simulink model "EPD629_WilliamsJ_Project_"  (R2021b)
settings: Solver=VariableStepAuto  StartTime=0.0  StopTime=StopTime  MaxStep=0.005  RelTol=1e-4
values from neighbouring files (symbols this model uses):
  AxleRatio = 11.47    [ProjectScript.m]
  BrakeDrag_N = 2.5    [ProjectScript.m]
  CableStrokeVsPedalPos_mmpdeg = 0.995519    [ProjectScript.m]
  Cd = 0.7691142    [ProjectScript.m]
  Crr = 0.0138796    [ProjectScript.m]
  CTireRollRadius = 0.944    [ProjectScript.m]
  CVTEngagementSpd_rpm = 1400    [ProjectScript.m]
  CVTRatioCoeffVsMphA = 0.000494471902965804    (= 0.000494471902966)    [ProjectScript.m]
  CVTRatioCoeffVsMphB = -0.0203171948865201    (= -0.0203171948865)    [ProjectScript.m]
  CVTRatioCoeffVsMphC = 0.301637634575451    (= 0.301637634575)    [ProjectScript.m]
  CVTRatioCoeffVsMphD = -2.09463337350964    (= -2.09463337351)    [ProjectScript.m]
  CVTRatioCoeffVsMphE = 7.47628950179633    (= 7.4762895018)    [ProjectScript.m]
  DistCableSinkThrottle_mm = 0.25    [ProjectScript.m]
  EngPowerTableData_hp = [0, 0, 0, 0, 0 ... (first row only)    [ProjectScript.m]
  EngPowerTableSpdBreakpoints_rpm = (0:500:7500)    [ProjectScript.m]
  EngPowerTableThrottleBreakpoints_prcnt = [0:.25:1]    [ProjectScript.m]
  FlyCoeffAClosed = 5.31512605042017e-8    (= 5.31512605042e-08)    [ProjectScript.m]
  FlyCoeffAOpen = 2.27450980392157e-7    (= 2.27450980392e-07)    [ProjectScript.m]
  FlyCoeffBClosed = 0.0000162815126050419    (= 1.6281512605e-05)    [ProjectScript.m]
  FlyCoeffBOpen = -0.000070868347338936    (= -7.08683473389e-05)    [ProjectScript.m]
  FlyCoeffCClosed = -0.0102941176470588    (= -0.0102941176471)    [ProjectScript.m]
  FlyCoeffCOpen = 0.00588235294117689    (= 0.00588235294118)    [ProjectScript.m]
  g = 9.80665    [ProjectScript.m]
  GearboxRatio = 1.95    [ProjectScript.m]
  GovArmRange_deg = 14.7    [ProjectScript.m]
  GradeIncline_pcnt = 0    [ProjectScript.m]
  LengthGovArmLower_mm = 90.4    [ProjectScript.m]
  LengthGovArmUpper_mm = 67.5    [ProjectScript.m]
  MassVehicle_kg = (CurbWeight_lbm + VehiclePayload_lbm)*0.4535924    (= 589.67012)    [ProjectScript.m]
  PedalPosMax_deg = 30    [ProjectScript.m]
  PedalTravelIntTension_deg = 10    [ProjectScript.m]
  rho_air = 1.224991    [ProjectScript.m]
  SpringRate_lbfpin = 12.6    [ProjectScript.m]
  ThrottleCableDia_mm = 1.190625    [ProjectScript.m]
  ThrottleLeverArmRadius_mm = 14.25    [ProjectScript.m]
  ThrottlePosMax_deg = 82    [ProjectScript.m]
  ThrottleReturnSpringPreload_Nmm = 163.7711    [ProjectScript.m]
  ThrottleReturnSpringRate_Nmmpdeg = 0.786881    [ProjectScript.m]
  TireDia_in = 18    [ProjectScript.m]
  VehicleFrontalArea_m2 = 1.8    [ProjectScript.m]
undefined symbols (not defined in the file or in its folder): CaptureTime, DesCruisingSpeed_mph, GovernorSet, Pedal_Change_After_Dyno
libraries: simulink x7, simulink_extras x2
settings Model: Creator=jwilli42  LastModifiedBy=jwilli42
settings OptimizationCC: BlockReduction=off  DefaultParameterBehavior=Inlined  BufferReuse=off
settings DebuggingCC: AlgebraicLoopMsg=none

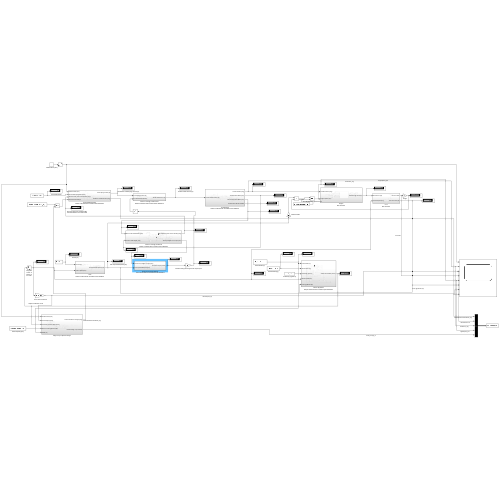
[thumbnail: Simulink's stored preview of the top-level diagram]
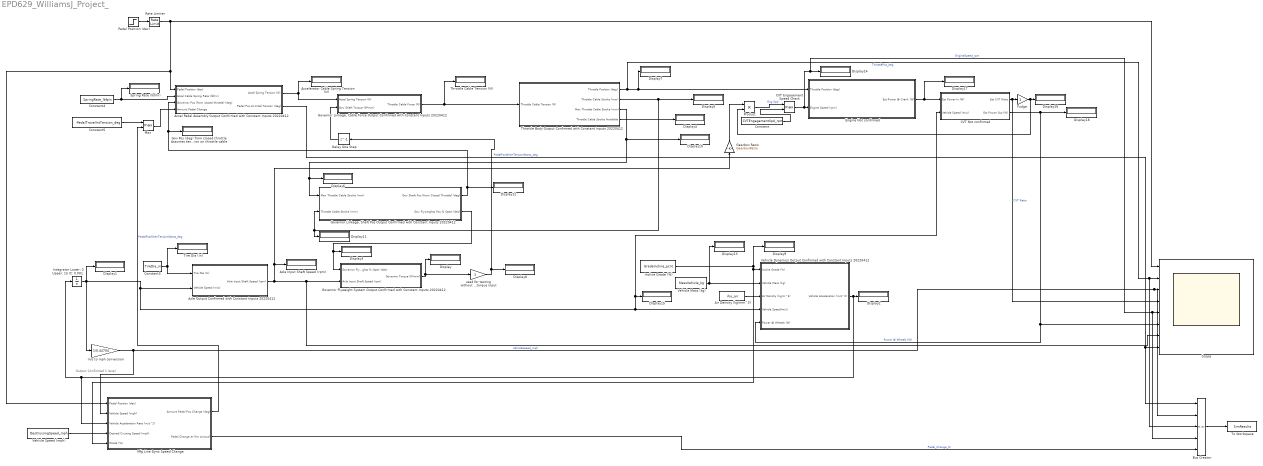
== system EPD629_WilliamsJ_Project_ ==
  note: Output Confirmed 1 level
  Accel Pedal Assembly Output Confirmed with Constant Inputs 20220412 : Subsystem
  Accelerator Cable Spring Tension (N) : Display
  Air Density (kg/mm^3) : Constant  Value=rho_air
  Axle Output Confirmed with Constant Inputs 20220412 : Subsystem
  Axle Input Shaft Speed (rpm) : Display
  Bus Creator : BusCreator  Inputs=5
  CVT Not confirmed : Subsystem
  CVT Engagement Speed Check : MinMax  Function=max  Inputs=2
  Constant : Constant  Value=CVTEngagementSpd_rpm
  Constant3 : Constant  Value=TireDia_in
  Constant4 : Constant  Value=SpringRate_lbfpin
  Constant5 : Constant  Value=-PedalTravelIntTension_deg
  Delay One Step : Delay  DelayLength=1
  Display{,1..18} (19 alike) : Display
  Engine Not confirmed : Subsystem
  Fudge : Gain
  Gearbox Ratio : Gain  Gain=GearboxRatio
  Gov Pos (deg) from closed throttle Assumes tension on throttle cable : Display
  Governor Flyweight System Output Confirmed with Constant Inputs 20220412 : Subsystem
  "Governor Linkage, Cable Force Output Confirmed with Constant Inputs 20220412" : Subsystem
  "Governor Linkage, Shaft Pos Output Confirmed with Constant Inputs 20220412" : Subsystem
  Incline Grade (%) : Constant  Value=GradeIncline_pcnt
  "Integrator Lower: 0 Upper: 15 IC: 0.001 " : Integrator  InitialCondition=.1  LimitOutput=on  UpperSaturationLimit=15  LowerSaturationLimit=0
  Max : MinMax  Function=max  Inputs=2
  Mfg Line Dyno Speed Change : Subsystem
  Pedal Position (dec) : Step  Time=0.5  SampleTime=0
  Product : Product
  Rate Limiter : RateLimiter  RisingSlewLimit=20  FallingSlewLimit=-30  SampleTimeMode=inherited
  Scope : Scope  NumInputPorts=8
  Spring Rate (lbf/in) : Display
  Throttle Body Output Confirmed with Constant Inputs 20220412 : Subsystem
  "Throttle Cable Tension (N) " : Display
  Tire Dia (in) : Display
  To Workspace : ToWorkspace  VariableName=SimResults  SaveFormat=Timeseries  SampleTime=-1
      settings: MaxDataPoints=1
  "Vehicle Dynamics Output Confirmed with Constant Inputs 20220412 " : Subsystem
  Vehicle Mass (kg) : Constant  Value=MassVehicle_kg
  Vehicle Speed (mph) : Constant  Value=DesCruisingSpeed_mph
  m/s to mph conversion : Gain  Gain=1/0.44704
  used for testing without governor torque input : Gain
  wires:
  Vehicle Mass (kg)/1 -> "Vehicle Dynamics Output Confirmed with Constant Inputs 20220412 "/2(Vehicle Mass (kg)), Display13/1
  Air Density (kg/mm^3)/1 -> "Vehicle Dynamics Output Confirmed with Constant Inputs 20220412 "/3(Air Density (kg/m^3))
  Vehicle Speed (mph)/1 -> Mfg Line Dyno Speed Change/4(Desired Cruising Speed (mph))
  Constant3/1 -> Tire Dia (in)/1, Axle Output Confirmed with Constant Inputs 20220412/1(Tire Dia (In))
  Throttle Body Output Confirmed with Constant Inputs 20220412/3(Max Throttle Cable Stroke (mm)) -> Display10/1, "Governor Linkage, Shaft Pos Output Confirmed with Constant Inputs 20220412"/1(Max Throttle Cable Stroke (mm)), Display6/1
  Axle Output Confirmed with Constant Inputs 20220412/1(Axle Input Shaft Speed (rpm)) -> Axle Input Shaft Speed (rpm)/1, Gearbox Ratio/1, Scope/7, Governor Flyweight System Output Confirmed with Constant Inputs 20220412/2(Axle Input Shaft Speed (rpm))
  Constant4/1 -> Accel Pedal Assembly Output Confirmed with Constant Inputs 20220412/2(Accel Cable Spring Rate (lbf/in)), Spring Rate (lbf/in)/1
  Pedal Position (dec)/1 -> Rate Limiter/1
  Throttle Body Output Confirmed with Constant Inputs 20220412/1(Throttle Position (deg)) -> Scope/2, Bus Creator/3, Engine Not confirmed/1(Throttle Position (deg)), Display7/1  "ThrottlePos_deg"
  Throttle Body Output Confirmed with Constant Inputs 20220412/4(Throttle Cable Stroke Available) -> Display4/1
  Engine Not confirmed/1(Est Power @ Crank (W)) -> Display17/1, CVT Not confirmed/1(Est Power In (W))
  Gearbox Ratio/1 -> Product/1
  CVT Not confirmed/1(Est CVT Ratio) -> Scope/4, Fudge/1  "CVT Ratio"
  Fudge/1 -> Display16/1, Product/2
  CVT Not confirmed/2(Est Power Out (W)) -> "Vehicle Dynamics Output Confirmed with Constant Inputs 20220412 "/5(Power @ Wheels (W)), Scope/6, Display18/1  "Power @ Wheels (W)"
  m/s to mph conversion/1 -> Bus Creator/2, Scope/3, Mfg Line Dyno Speed Change/2(Vehicle Speed (mph))  "VehicleSpeed_mph"
  Product/1 -> CVT Engagement Speed Check/1  "Eng Spd"
  Constant/1 -> CVT Engagement Speed Check/2
  Governor Flyweight System Output Confirmed with Constant Inputs 20220412/1(Governor Torque (N*mm)) -> Display/1, used for testing without governor torque input/1
  CVT Engagement Speed Check/1 -> Scope/5, Bus Creator/4, Display14/1, Engine Not confirmed/2(Engine Speed (rpm))  "EngineSpeed_rpm"
  Rate Limiter/1 -> Mfg Line Dyno Speed Change/1(Pedal Position (dec)), Accel Pedal Assembly Output Confirmed with Constant Inputs 20220412/1(Pedal Position (dec)), Scope/1
  Mfg Line Dyno Speed Change/1(Amount Pedal Pos Change (deg)) -> Max/2  "PedalPosWhenTensionStarts_deg"
  Incline Grade (%)/1 -> Mfg Line Dyno Speed Change/5(Grade (%)), "Vehicle Dynamics Output Confirmed with Constant Inputs 20220412 "/1(Incline Grade (%)), Display9/1
  Constant5/1 -> Max/1
  Max/1 -> Accel Pedal Assembly Output Confirmed with Constant Inputs 20220412/4(Amount Pedal Change)
  Accel Pedal Assembly Output Confirmed with Constant Inputs 20220412/2(Pedal Pos at Initial Tension (deg)) -> Scope/8, Bus Creator/1  "PedalPosWhenTensionStarts_deg"
  Mfg Line Dyno Speed Change/2(Pedal Change Itr (for simout)) -> Bus Creator/5  "Pedal_Change_Itr"
  Bus Creator/1 -> To Workspace/1
  used for testing without governor torque input/1 -> Delay One Step/1, Display8/1
  "Vehicle Dynamics Output Confirmed with Constant Inputs 20220412 "/1(Vehicle Acceleration (m/s^2)) -> Mfg Line Dyno Speed Change/3(Vehicle Acceleration Rate (m/s^2)), "Integrator Lower: 0 Upper: 15 IC: 0.001 "/1, Display2/1
  Delay One Step/1 -> "Governor Linkage, Cable Force Output Confirmed with Constant Inputs 20220412"/2(Gov Shaft Torque (N*mm))
  Accel Pedal Assembly Output Confirmed with Constant Inputs 20220412/1(Accel Spring Tension (N)) -> "Governor Linkage, Cable Force Output Confirmed with Constant Inputs 20220412"/1(Accel Spring Tension (N)), Accelerator Cable Spring Tension (N)/1
  "Integrator Lower: 0 Upper: 15 IC: 0.001 "/1 -> m/s to mph conversion/1, CVT Not confirmed/2(Vehicle Speed (m/s)), Display15/1, "Vehicle Dynamics Output Confirmed with Constant Inputs 20220412 "/4(Vehicle Speed(m/s)), Axle Output Confirmed with Constant Inputs 20220412/2(Vehicle Speed (m/s)), Display1/1
  "Governor Linkage, Shaft Pos Output Confirmed with Constant Inputs 20220412"/2(Gov Flyweights Pos % Open (dec)) -> Governor Flyweight System Output Confirmed with Constant Inputs 20220412/1(Governor Flyweights % Open (dec)), Display3/1
  "Governor Linkage, Cable Force Output Confirmed with Constant Inputs 20220412"/1(Throttle Cable Force (N)) -> Throttle Body Output Confirmed with Constant Inputs 20220412/1(Throttle Cable Tension (N)), "Throttle Cable Tension (N) "/1
  "Governor Linkage, Shaft Pos Output Confirmed with Constant Inputs 20220412"/1(Gov Shaft Pos (from Closed Throttle) (deg)) -> Accel Pedal Assembly Output Confirmed with Constant Inputs 20220412/3(Governor Pos (from closed throttle) (deg)), Gov Pos (deg) from closed throttle Assumes tension on throttle cable/1, Display12/1
  Throttle Body Output Confirmed with Constant Inputs 20220412/2(Throttle Cable Stroke (mm)) -> "Governor Linkage, Shaft Pos Output Confirmed with Constant Inputs 20220412"/2(Throttle Cable Stroke (mm)), Display11/1, Display5/1

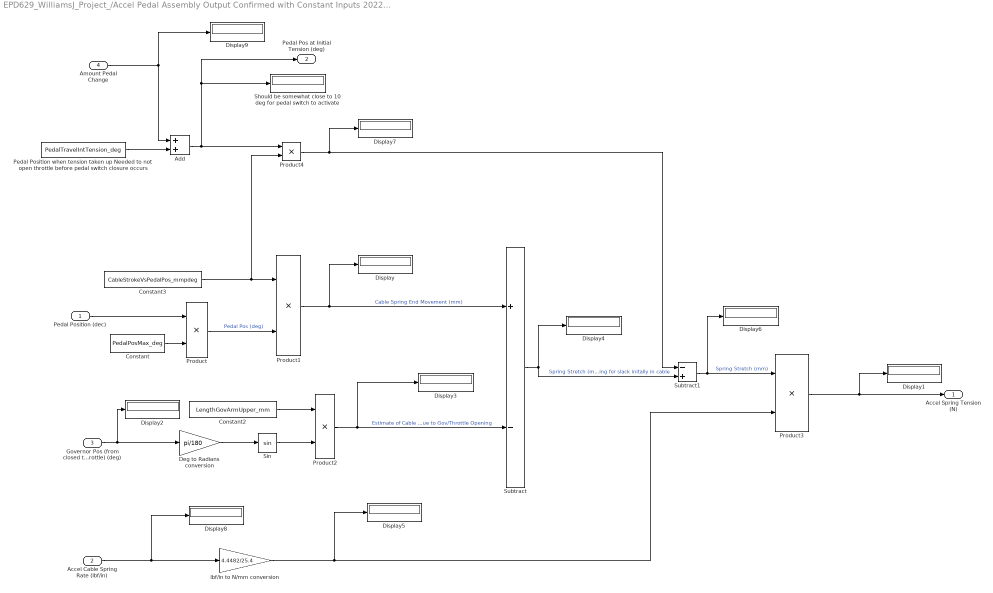
== system EPD629_WilliamsJ_Project_/Accel Pedal Assembly Output Confirmed with Constant Inputs 20220412 ==
  Pedal Position (dec) : Inport
  Accel Cable Spring Rate (lbf/in) : Inport  Port=2
  Governor Pos (from closed throttle) (deg) : Inport  Port=3
  Amount Pedal Change : Inport  Port=4
  Add : Sum
  Constant : Constant  Value=PedalPosMax_deg
  Constant2 : Constant  Value=LengthGovArmUpper_mm
  Constant3 : Constant  Value=CableStrokeVsPedalPos_mmpdeg
  Deg to Radians conversion : Gain  Gain=pi/180
  Display{,1..9} (10 alike) : Display
  Pedal Position when tension taken up Needed to not open throttle before pedal switch closure occurs : Constant  Value=PedalTravelIntTension_deg
  Product{,1..4} (5 alike) : Product
  Should be somewhat close to 10 deg for pedal switch to activate : Display
  Sin : Trigonometry
  Subtract : Sum  Inputs=+-
  Subtract1 : Sum  Inputs=-+
  lbf/in to N/mm conversion : Gain  Gain=4.4482/25.4
  Accel Spring Tension (N) : Outport
  Pedal Pos at Initial Tension (deg) : Outport  Port=2
  wires:
  Constant/1 -> Product/2
  Product/1 -> Product1/2  "Pedal Pos (deg)"
  Governor Pos (from closed throttle) (deg)/1 -> Display2/1, Deg to Radians conversion/1
  Deg to Radians conversion/1 -> Sin/1
  Sin/1 -> Product2/2
  Constant2/1 -> Product2/1
  Product1/1 -> Display/1, Subtract/1  "Cable Spring End Movement (mm)"
  Product2/1 -> Display3/1, Subtract/2  "Estimate of Cable Travel Due to Gov/Throttle Opening"
  lbf/in to N/mm conversion/1 -> Display5/1, Product3/2
  Subtract/1 -> Subtract1/2, Display4/1  "Spring Stretch (mm) w/out accounting for slack initally in cable"
  Product3/1 -> Display1/1, Accel Spring Tension (N)/1
  Accel Cable Spring Rate (lbf/in)/1 -> Display8/1, lbf/in to N/mm conversion/1
  Product4/1 -> Subtract1/1, Display7/1
  Subtract1/1 -> Product3/1, Display6/1  "Spring Stretch (mm)"
  Pedal Position (dec)/1 -> Product/1
  Pedal Position when tension taken up Needed to not open throttle before pedal switch closure occurs/1 -> Add/2
  Constant3/1 -> Product1/1, Product4/2
  Add/1 -> Pedal Pos at Initial Tension (deg)/1, Should be somewhat close to 10 deg for pedal switch to activate/1, Product4/1
  Amount Pedal Change/1 -> Add/1, Display9/1

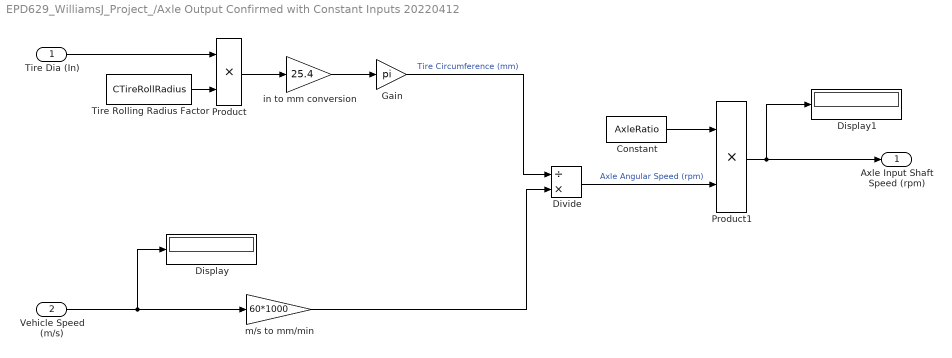
== system EPD629_WilliamsJ_Project_/Axle Output Confirmed with Constant Inputs 20220412 ==
  Tire Dia (In) : Inport
  Vehicle Speed (m/s) : Inport  Port=2
  Constant : Constant  Value=AxleRatio
  Display : Display
  Display1 : Display
  Divide : Product  Inputs=/*
  Gain : Gain  Gain=pi
  Product : Product
  Product1 : Product
  Tire Rolling Radius Factor : Constant  Value=CTireRollRadius
  in to mm conversion : Gain  Gain=25.4
  m/s to mm/min : Gain  Gain=60*1000
  Axle Input Shaft Speed (rpm) : Outport
  wires:
  Tire Rolling Radius Factor/1 -> Product/2
  Tire Dia (In)/1 -> Product/1
  Product/1 -> in to mm conversion/1
  in to mm conversion/1 -> Gain/1
  Gain/1 -> Divide/1  "Tire Circumference (mm)"
  Vehicle Speed (m/s)/1 -> Display/1, m/s to mm/min/1
  m/s to mm/min/1 -> Divide/2
  Divide/1 -> Product1/2  "Axle Angular Speed (rpm)"
  Constant/1 -> Product1/1
  Product1/1 -> Display1/1, Axle Input Shaft Speed (rpm)/1

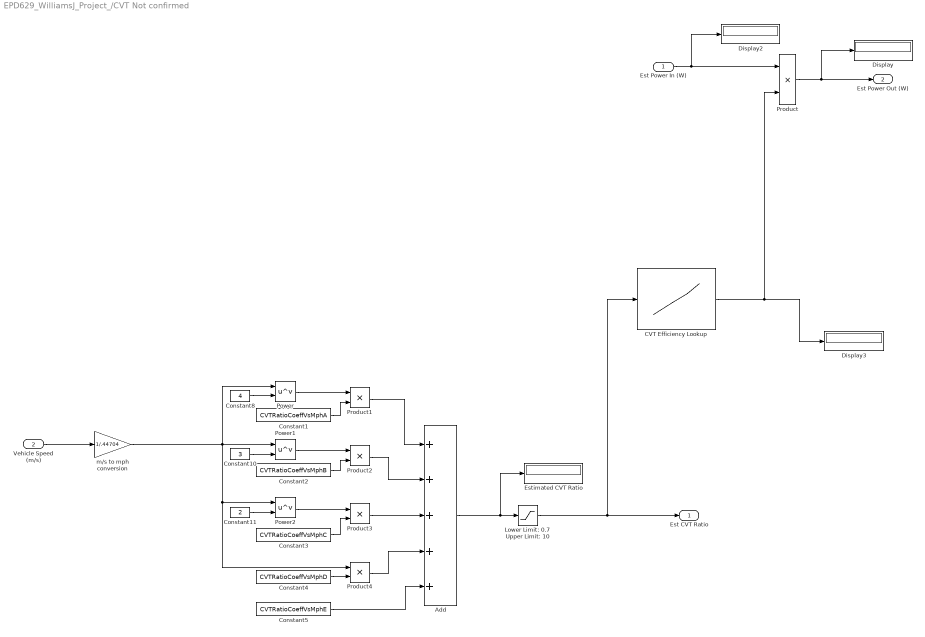
== system EPD629_WilliamsJ_Project_/CVT Not confirmed ==
  Est Power In (W) : Inport
  Vehicle Speed (m/s) : Inport  Port=2
  Add : Sum  Inputs=+++++
  CVT Efficiency Lookup : Lookup_n-D  NumberOfTableDimensions=1  BreakpointsForDimension1=[0.7, 0.8, 0.9, 1.1, 1.5, 1.75, 1.9, 2.1, 2.3]  Table=[0.35, 0.48, 0.57, 0.63, 0.68, 0.62, 0.59, 0.58, 0.6]  ExtrapMethod=Clip  UseLastTableValue=on  InternalRulePriority=Speed  RndMeth=Simplest  InputSameDT=on
  Constant1 : Constant  Value=CVTRatioCoeffVsMphA
  Constant10 : Constant  Value=3
  Constant11 : Constant  Value=2
  Constant2 : Constant  Value=CVTRatioCoeffVsMphB
  Constant3 : Constant  Value=CVTRatioCoeffVsMphC
  Constant4 : Constant  Value=CVTRatioCoeffVsMphD
  Constant5 : Constant  Value=CVTRatioCoeffVsMphE
  Constant8 : Constant  Value=4
  Display : Display
  Display2 : Display
  Display3 : Display
  Estimated CVT Ratio : Display
  Lower Limit: 0.7 Upper Limit: 10 : Saturate  UpperLimit=10  LowerLimit=0.7
  Power : Math  Operator=pow  SaturateOnIntegerOverflow=on
  Power1 : Math  Operator=pow  SaturateOnIntegerOverflow=on
  Power2 : Math  Operator=pow  SaturateOnIntegerOverflow=on
  Product{,1..4} (5 alike) : Product
  m/s to mph conversion : Gain  Gain=1/.44704
  Est CVT Ratio : Outport
  Est Power Out (W) : Outport  Port=2
  wires:
  Est Power In (W)/1 -> Display2/1, Product/1
  Product/1 -> Display/1, Est Power Out (W)/1
  Constant8/1 -> Power/2
  Power/1 -> Product1/1
  Constant1/1 -> Product1/2
  Constant10/1 -> Power1/2
  Constant11/1 -> Power2/2
  m/s to mph conversion/1 -> Power/1, Product4/1, Power2/1, Power1/1
  Power1/1 -> Product2/1
  Constant2/1 -> Product2/2
  Power2/1 -> Product3/1
  Constant3/1 -> Product3/2
  Constant4/1 -> Product4/2
  Product3/1 -> Add/3
  Product2/1 -> Add/2
  Product1/1 -> Add/1
  Product4/1 -> Add/4
  Constant5/1 -> Add/5
  Add/1 -> Lower Limit: 0.7 Upper Limit: 10/1, Estimated CVT Ratio/1
  Vehicle Speed (m/s)/1 -> m/s to mph conversion/1
  Lower Limit: 0.7 Upper Limit: 10/1 -> Est CVT Ratio/1, CVT Efficiency Lookup/1
  CVT Efficiency Lookup/1 -> Display3/1, Product/2

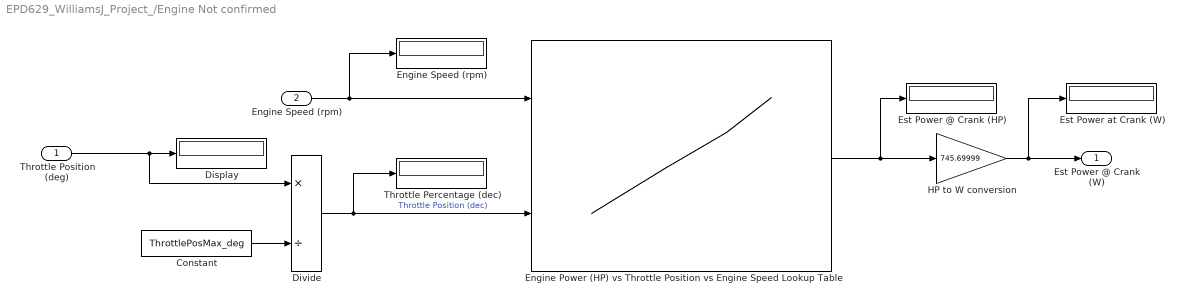
== system EPD629_WilliamsJ_Project_/Engine Not confirmed ==
  Throttle Position (deg) : Inport
  Engine Speed (rpm) : Inport  Port=2
  Constant : Constant  Value=ThrottlePosMax_deg
  Display : Display
  Divide : Product  Inputs=*/
  Engine Power (HP) vs Throttle Position vs Engine Speed Lookup Table : Lookup_n-D  BreakpointsForDimension1=EngPowerTableSpdBreakpoints_rpm  BreakpointsForDimension2=EngPowerTableThrottleBreakpoints_prcnt  Table=EngPowerTableData_hp  InternalRulePriority=Speed  RndMeth=Simplest  InputSameDT=on
      settings: InputPortMap=u0,u1
  "Engine Speed (rpm) " : Display
  Est Power @ Crank (HP) : Display
  Est Power at Crank (W) : Display
  HP to W conversion : Gain  Gain=745.69999
  Throttle Percentage (dec) : Display
  Est Power @ Crank (W) : Outport
  wires:
  Constant/1 -> Divide/2
  Divide/1 -> Engine Power (HP) vs Throttle Position vs Engine Speed Lookup Table/2, Throttle Percentage (dec)/1  "Throttle Position (dec)"
  Throttle Position (deg)/1 -> Display/1, Divide/1
  Engine Power (HP) vs Throttle Position vs Engine Speed Lookup Table/1 -> Est Power @ Crank (HP)/1, HP to W conversion/1
  HP to W conversion/1 -> Est Power at Crank (W)/1, Est Power @ Crank (W)/1
  Engine Speed (rpm)/1 -> "Engine Speed (rpm) "/1, Engine Power (HP) vs Throttle Position vs Engine Speed Lookup Table/1

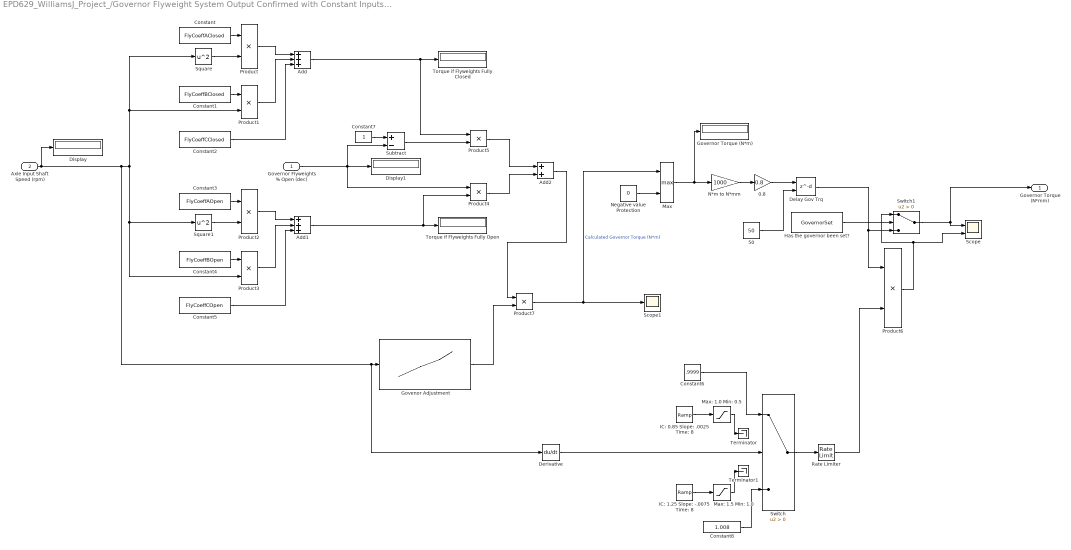
== system EPD629_WilliamsJ_Project_/Governor Flyweight System Output Confirmed with Constant Inputs 20220412 ==
  Governor Flyweights % Open (dec) : Inport
  Axle Input Shaft Speed (rpm) : Inport  Port=2
  0.8 : Gain  Gain=0.8
  50 : Constant  Value=50
  Add : Sum  Inputs=+++
  Add1 : Sum  Inputs=+++
  Add2 : Sum
  Constant : Constant  Value=FlyCoeffAClosed
  Constant1 : Constant  Value=FlyCoeffBClosed
  Constant2 : Constant  Value=FlyCoeffCClosed
  Constant3 : Constant  Value=FlyCoeffAOpen
  Constant4 : Constant  Value=FlyCoeffBOpen
  Constant5 : Constant  Value=FlyCoeffCOpen
  Constant6 : Constant  Value=.9999
  Constant7 : Constant
  Constant8 : Constant  Value=1.008
  Delay Gov Trq : Delay  DelayLengthSource=Input port  DelayLengthUpperLimit=5000
      settings: InputPortMap=u0,p1
  Derivative : Derivative
  Display : Display
  Display1 : Display
  Govenor Adjustment : Lookup_n-D  NumberOfTableDimensions=1  BreakpointsForDimension1=[0, 500, 1000, 1250, 1500, 2000, 2500, 3000, 3500, 4000]  Table=[0.7, .75, 0.9, 1.2, 1.5, 1.75, 1.75, 1.75, 1.75 1.75]  ExtrapMethod=Clip  UseLastTableValue=on  InternalRulePriority=Speed  RndMeth=Simplest  InputSameDT=on
  Governor Torque (N*m) : Display
  Has the governor been set? : Constant  Value=GovernorSet
  IC: 0.85 Slope: .0025 Time: 8 : simulink/Sources/Ramp  slope=.0025  start=8  InitialOutput=.5
  IC: 1.25 Slope: -.0075 Time: 8 : simulink/Sources/Ramp  slope=-.0075  start=8  InitialOutput=1.05
  Max : MinMax  Function=max  Inputs=2
  Max: 1.0 Min: 0.5 : Saturate  UpperLimit=.9  LowerLimit=.5
  Max: 1.5 Min: 1.0 : Saturate  UpperLimit=1.5  LowerLimit=1.1
  N*m to N*mm : Gain  Gain=1000
  Negative value Protection : Constant  Value=0
  Product{,1..7} (8 alike) : Product
  Rate Limiter : RateLimiter  RisingSlewLimit=.1  FallingSlewLimit=-.1  SampleTimeMode=inherited
  Scope : Scope  NumInputPorts=2
  Scope1 : Scope
  Square : Math  Operator=square  SaturateOnIntegerOverflow=on
  Square1 : Math  Operator=square  SaturateOnIntegerOverflow=on
  Subtract : Sum  Inputs=+-
  Switch : Switch  Criteria=u2 > Threshold
  Switch1 : Switch  Criteria=u2 > Threshold
  Terminator : Terminator
  Terminator1 : Terminator
  Torque if Flyweights Fully Closed : Display
  Torque if Flyweights Fully Open : Display
  Governor Torque (N*mm) : Outport
  wires:
  Axle Input Shaft Speed (rpm)/1 -> Derivative/1, Govenor Adjustment/1, Product1/2, Square/1, Square1/1, Product3/2, Display/1
  Product/1 -> Add/1
  Product1/1 -> Add/2
  Constant2/1 -> Add/3
  Constant1/1 -> Product1/1
  Constant/1 -> Product/1
  Square/1 -> Product/2
  Square1/1 -> Product2/2
  Constant3/1 -> Product2/1
  Constant4/1 -> Product3/1
  Constant5/1 -> Add1/3
  Product3/1 -> Add1/2
  Product2/1 -> Add1/1
  N*m to N*mm/1 -> 0.8/1
  Negative value Protection/1 -> Max/2
  Max/1 -> Governor Torque (N*m)/1, N*m to N*mm/1
  Add2/1 -> Product7/1
  Constant7/1 -> Subtract/1
  Governor Flyweights % Open (dec)/1 -> Display1/1, Subtract/2, Product4/1
  Add1/1 -> Torque if Flyweights Fully Open/1, Product4/2
  Product4/1 -> Add2/2
  Subtract/1 -> Product5/2
  Add/1 -> Torque if Flyweights Fully Closed/1, Product5/1
  Product5/1 -> Add2/1
  0.8/1 -> Delay Gov Trq/1
  Delay Gov Trq/1 -> Switch1/3, Product6/1
  50/1 -> Delay Gov Trq/2
  IC: 0.85 Slope: .0025 Time: 8/1 -> Max: 1.0 Min: 0.5/1
  IC: 1.25 Slope: -.0075 Time: 8/1 -> Max: 1.5 Min: 1.0/1
  Switch/1 -> Rate Limiter/1
  Switch1/1 -> Scope/1, Governor Torque (N*mm)/1
  Product6/1 -> Scope/2, Switch1/1
  Product7/1 -> Max/1, Scope1/1  "Calculated Governor Torque (N*m)"
  Rate Limiter/1 -> Product6/2
  Constant8/1 -> Switch/3
  Constant6/1 -> Switch/1
  Has the governor been set?/1 -> Switch1/2
  Max: 1.0 Min: 0.5/1 -> Terminator/1
  Max: 1.5 Min: 1.0/1 -> Terminator1/1
  Derivative/1 -> Switch/2
  Govenor Adjustment/1 -> Product7/2

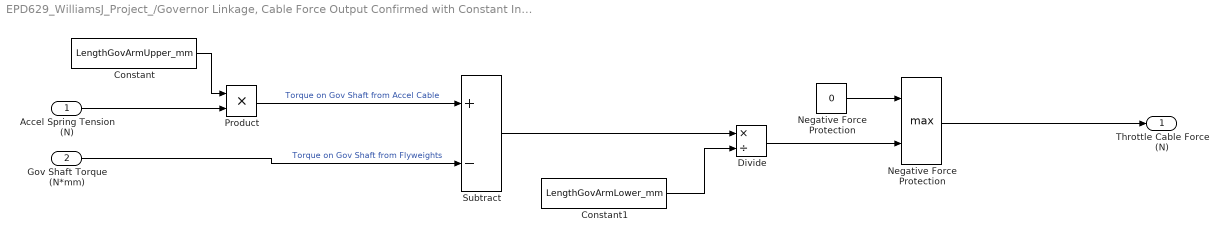
== system EPD629_WilliamsJ_Project_/Governor Linkage, Cable Force Output Confirmed with Constant Inputs 20220412 ==
  Accel Spring Tension (N) : Inport
  Gov Shaft Torque (N*mm) : Inport  Port=2
  Constant : Constant  Value=LengthGovArmUpper_mm
  Constant1 : Constant  Value=LengthGovArmLower_mm
  Divide : Product  Inputs=*/
  Negative Force Protection : Constant  Value=0
  "Negative Force Protection " : MinMax  Function=max  Inputs=2
  Product : Product
  Subtract : Sum  Inputs=+-
  Throttle Cable Force (N) : Outport
  wires:
  Accel Spring Tension (N)/1 -> Product/2
  Constant/1 -> Product/1
  Product/1 -> Subtract/1  "Torque on Gov Shaft from Accel Cable"
  Gov Shaft Torque (N*mm)/1 -> Subtract/2  "Torque on Gov Shaft from Flyweights"
  Subtract/1 -> Divide/1
  Constant1/1 -> Divide/2
  Divide/1 -> "Negative Force Protection "/2
  Negative Force Protection/1 -> "Negative Force Protection "/1
  "Negative Force Protection "/1 -> Throttle Cable Force (N)/1

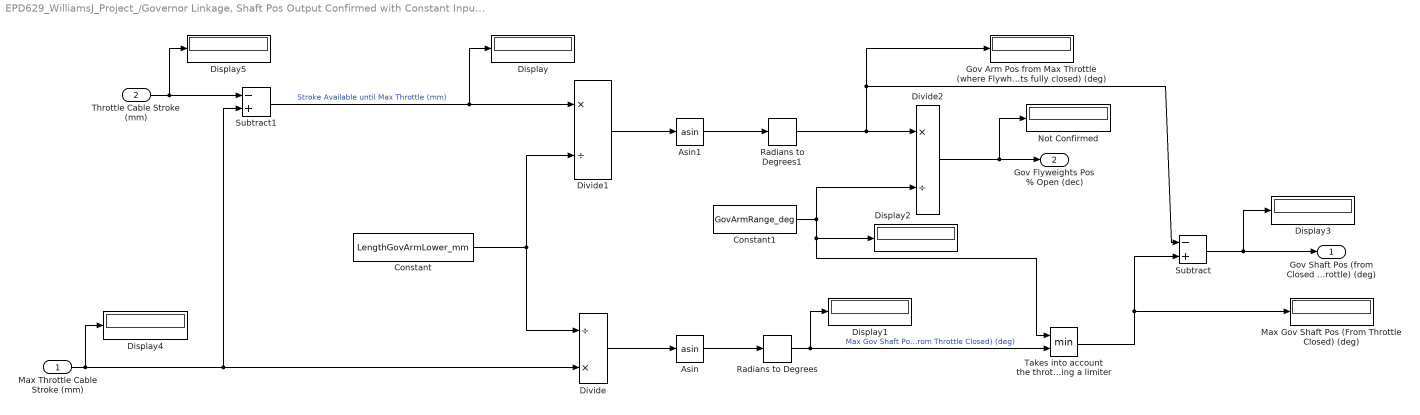
== system EPD629_WilliamsJ_Project_/Governor Linkage, Shaft Pos Output Confirmed with Constant Inputs 20220412 ==
  Max Throttle Cable Stroke (mm) : Inport
  Throttle Cable Stroke (mm) : Inport  Port=2
  Asin : Trigonometry  Operator=asin
  Asin1 : Trigonometry  Operator=asin
  Constant : Constant  Value=LengthGovArmLower_mm
  Constant1 : Constant  Value=GovArmRange_deg
  Display{,1..5} (6 alike) : Display
  Divide : Product  Inputs=/*
  Divide1 : Product  Inputs=*/
  Divide2 : Product  Inputs=*/
  Gov Arm Pos from Max Throttle (where Flywheights fully closed) (deg) : Display
  Max Gov Shaft Pos (From Throttle Closed) (deg) : Display
  Not Confirmed : Display
  Radians to Degrees : simulink_extras/Transformations/Radians to Degrees
  Radians to Degrees1 : simulink_extras/Transformations/Radians to Degrees
  Subtract : Sum  Inputs=-+
  Subtract1 : Sum  Inputs=-+
  Takes into account the throttle stop OR the governor shaft stop being a limiter : MinMax  Inputs=2
  Gov Shaft Pos (from Closed Throttle) (deg) : Outport
  Gov Flyweights Pos % Open (dec) : Outport  Port=2
  wires:
  Max Throttle Cable Stroke (mm)/1 -> Display4/1, Subtract1/2, Divide/2
  Divide/1 -> Asin/1
  Asin/1 -> Radians to Degrees/1
  Radians to Degrees/1 -> Takes into account the throttle stop OR the governor shaft stop being a limiter/2, Display1/1  "Max Gov Shaft Pos (From Throttle Closed) (deg)"
  Constant/1 -> Divide1/2, Divide/1
  Divide1/1 -> Asin1/1
  Asin1/1 -> Radians to Degrees1/1
  Radians to Degrees1/1 -> Gov Arm Pos from Max Throttle (where Flywheights fully closed) (deg)/1, Subtract/1, Divide2/1
  Divide2/1 -> Not Confirmed/1, Gov Flyweights Pos % Open (dec)/1
  Constant1/1 -> Divide2/2, Display2/1, Takes into account the throttle stop OR the governor shaft stop being a limiter/1
  Takes into account the throttle stop OR the governor shaft stop being a limiter/1 -> Subtract/2, Max Gov Shaft Pos (From Throttle Closed) (deg)/1
  Subtract/1 -> Display3/1, Gov Shaft Pos (from Closed Throttle) (deg)/1
  Subtract1/1 -> Divide1/1, Display/1  "Stroke Available until Max Throttle (mm)"
  Throttle Cable Stroke (mm)/1 -> Subtract1/1, Display5/1

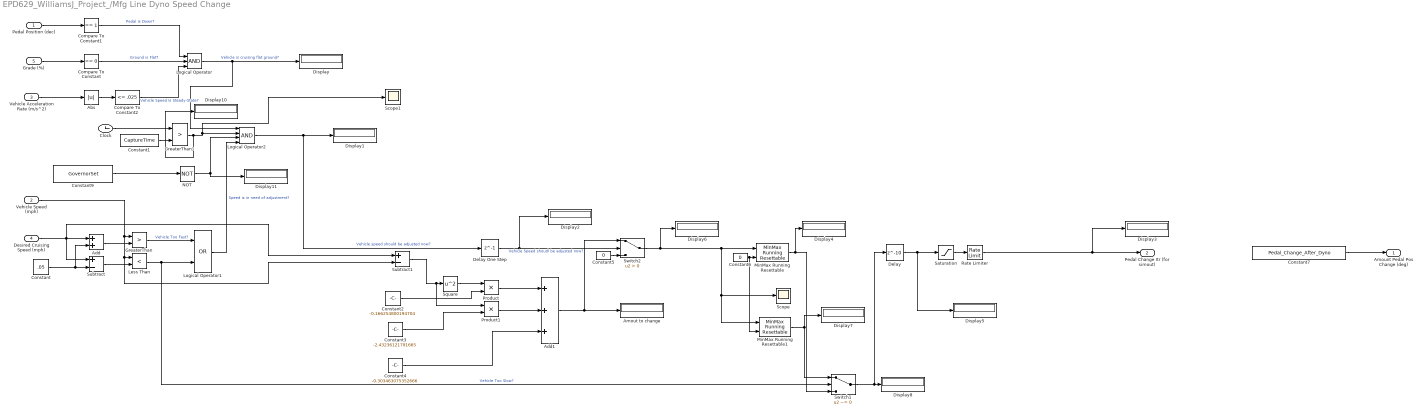
== system EPD629_WilliamsJ_Project_/Mfg Line Dyno Speed Change ==
  Pedal Position (dec) : Inport
  Vehicle Speed (mph) : Inport  Port=2
  Vehicle Acceleration Rate (m/s^2) : Inport  Port=3
  Desired Cruising Speed (mph) : Inport  Port=4
  Grade (%) : Inport  Port=5
  Abs : Abs
  Add : Sum
  Add1 : Sum  Inputs=+++
  Amout to change : Display
  Clock : Clock
  Compare To Constant : simulink/Logic and Bit Operations/Compare To Constant  relop===  const=0  OutDataTypeStr=boolean
  Compare To Constant1 : simulink/Logic and Bit Operations/Compare To Constant  relop===  const=1  OutDataTypeStr=boolean
  Compare To Constant2 : simulink/Logic and Bit Operations/Compare To Constant  relop=<=  const=.025  OutDataTypeStr=boolean
  Constant : Constant  Value=.05
  Constant1 : Constant  Value=CaptureTime
  Constant2 : Constant  Value=-0.166254800194704
  Constant3 : Constant  Value=-2.43236121791665
  Constant4 : Constant  Value=-0.303463075352666
  Constant5 : Constant  Value=0
  Constant6 : Constant  Value=0
  Constant7 : Constant  Value=Pedal_Change_After_Dyno
  Constant9 : Constant  Value=GovernorSet
  Delay : Delay  DelayLength=10
  Delay One Step : Delay  DelayLength=1
  Display{,1..8,10..11} (11 alike) : Display
  GreaterThan : RelationalOperator  Operator=>  OutDataTypeStr=boolean  RndMeth=Simplest
  GreaterThan1 : RelationalOperator  Operator=>  OutDataTypeStr=boolean  RndMeth=Simplest
  Less Than : RelationalOperator  Operator=<  OutDataTypeStr=boolean  RndMeth=Simplest
  Logical Operator : Logic  Inputs=3  AllPortsSameDT=off  OutDataTypeStr=boolean
  Logical Operator1 : Logic  Operator=OR  AllPortsSameDT=off  OutDataTypeStr=boolean
  Logical Operator2 : Logic  Inputs=4  AllPortsSameDT=off  OutDataTypeStr=boolean
  MinMax Running Resettable : simulink/Math Operations/MinMax Running Resettable  Function=max  vinit=0.0
  MinMax Running Resettable1 : simulink/Math Operations/MinMax Running Resettable  Function=min  vinit=0.0
  NOT : Logic  Operator=NOT  IconShape=distinctive  AllPortsSameDT=off  OutDataTypeStr=boolean
  Product : Product
  Product1 : Product
  Rate Limiter : RateLimiter  RisingSlewLimit=5  FallingSlewLimit=-5  SampleTimeMode=inherited
  Saturation : Saturate  UpperLimit=PedalPosMax_deg-PedalTravelIntTension_deg  LowerLimit=-PedalTravelIntTension_deg
  Scope : Scope
  Scope1 : Scope
  Square : Math  Operator=square  SaturateOnIntegerOverflow=on
  Subtract : Sum  Inputs=+-
  Subtract1 : Sum  Inputs=+-
  Switch1 : Switch  Criteria=u2 ~= 0
  Switch2 : Switch  Criteria=u2 > Threshold
  Amount Pedal Pos Change (deg) : Outport
  Pedal Change Itr (for simout) : Outport  Port=2
  wires:
  Logical Operator/1 -> Logical Operator2/1, Display/1  "Vehicle is cruising flat ground?"
  Pedal Position (dec)/1 -> Compare To Constant1/1
  Compare To Constant1/1 -> Logical Operator/1  "Pedal is Down?"
  Grade (%)/1 -> Compare To Constant/1
  Compare To Constant/1 -> Logical Operator/2  "Ground is Flat?"
  Vehicle Acceleration Rate (m/s^2)/1 -> Abs/1
  Abs/1 -> Compare To Constant2/1
  Compare To Constant2/1 -> Logical Operator/3  "Vehicle Speed Is Steady-State?"
  Vehicle Speed (mph)/1 -> Subtract1/2, Less Than/1, GreaterThan/1
  Desired Cruising Speed (mph)/1 -> Add/1, Subtract/1, Subtract1/1
  Constant/1 -> Add/2, Subtract/2
  Add/1 -> GreaterThan/2
  Subtract/1 -> Less Than/2
  GreaterThan/1 -> Logical Operator1/1  "Vehicle Too Fast?"
  Less Than/1 -> Switch1/2, Logical Operator1/2  "Vehicle Too Slow?"
  Logical Operator2/1 -> Display1/1, Delay One Step/1  "Vehicle speed should be adjusted now?"
  Subtract1/1 -> Product1/1, Square/1
  Square/1 -> Product/1
  Constant2/1 -> Product/2
  Product/1 -> Add1/1
  Product1/1 -> Add1/2
  Constant3/1 -> Product1/2
  Constant4/1 -> Add1/3
  Add1/1 -> Amout to change/1, Switch2/1
  Constant5/1 -> Switch2/3
  Switch2/1 -> Display6/1, Scope/1, MinMax Running Resettable1/1, MinMax Running Resettable/1
  Delay One Step/1 -> Display2/1, Switch2/2  "Vehicle Speed shoudl be adjusted now?"
  Constant6/1 -> MinMax Running Resettable1/2, MinMax Running Resettable/2
  MinMax Running Resettable/1 -> Switch1/3, Display4/1
  Delay/1 -> Saturation/1, Display5/1
  MinMax Running Resettable1/1 -> Switch1/1, Display7/1
  Saturation/1 -> Rate Limiter/1
  Switch1/1 -> Delay/1, Display8/1
  Rate Limiter/1 -> Display3/1, Pedal Change Itr (for simout)/1
  Constant7/1 -> Amount Pedal Pos Change (deg)/1
  Clock/1 -> GreaterThan1/1
  Constant1/1 -> GreaterThan1/2
  GreaterThan1/1 -> Display10/1, Scope1/1, Logical Operator2/2
  Logical Operator1/1 -> Logical Operator2/4  "Speed is in need of adjustment?"
  Constant9/1 -> NOT/1
  NOT/1 -> Display11/1, Logical Operator2/3

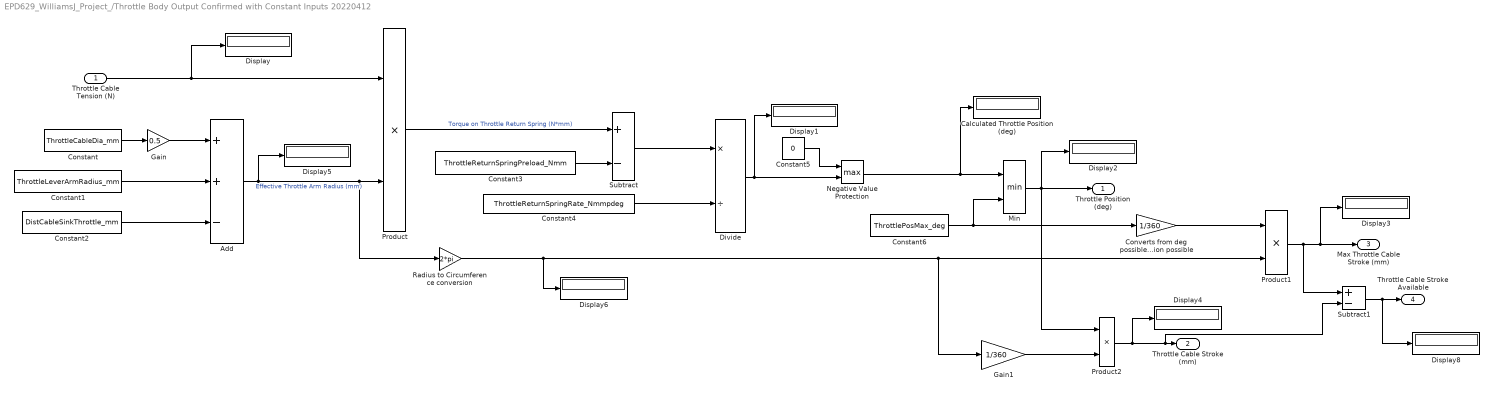
== system EPD629_WilliamsJ_Project_/Throttle Body Output Confirmed with Constant Inputs 20220412 ==
  Throttle Cable Tension (N) : Inport
  Add : Sum  Inputs=++-
  Calculated Throttle Position (deg) : Display
  Constant : Constant  Value=ThrottleCableDia_mm
  Constant1 : Constant  Value=ThrottleLeverArmRadius_mm
  Constant2 : Constant  Value=DistCableSinkThrottle_mm
  Constant3 : Constant  Value=ThrottleReturnSpringPreload_Nmm
  Constant4 : Constant  Value=ThrottleReturnSpringRate_Nmmpdeg
  Constant5 : Constant  Value=0
  Constant6 : Constant  Value=ThrottlePosMax_deg
  Converts from deg possible to percentage of rotation possible : Gain  Gain=1/360
  Display{,1..6,8} (8 alike) : Display
  Divide : Product  Inputs=*/
  Gain : Gain  Gain=0.5
  Gain1 : Gain  Gain=1/360
  Min : MinMax  Inputs=2
  Negative Value Protection : MinMax  Function=max  Inputs=2
  Product : Product
  Product1 : Product
  Product2 : Product
  Radius to Circumference conversion : Gain  Gain=2*pi
  Subtract : Sum  Inputs=+-
  Subtract1 : Sum  Inputs=+-
  Throttle Position (deg) : Outport
  Throttle Cable Stroke (mm) : Outport  Port=2
  Max Throttle Cable Stroke (mm) : Outport  Port=3
  Throttle Cable Stroke Available : Outport  Port=4
  wires:
  Constant/1 -> Gain/1
  Gain/1 -> Add/1
  Constant1/1 -> Add/2
  Constant2/1 -> Add/3
  Add/1 -> Display5/1, Product/2, Radius to Circumference conversion/1  "Effective Throttle Arm Radius (mm)"
  Product/1 -> Subtract/1  "Torque on Throttle Return Spring (N*mm)"
  Constant3/1 -> Subtract/2
  Subtract/1 -> Divide/1
  Constant4/1 -> Divide/2
  Constant5/1 -> Negative Value Protection/1
  Divide/1 -> Display1/1, Negative Value Protection/2
  Negative Value Protection/1 -> Calculated Throttle Position (deg)/1, Min/1
  Constant6/1 -> Min/2, Converts from deg possible to percentage of rotation possible/1
  Min/1 -> Display2/1, Throttle Position (deg)/1, Product2/1
  Converts from deg possible to percentage of rotation possible/1 -> Product1/1
  Radius to Circumference conversion/1 -> Product1/2, Gain1/1, Display6/1
  Product1/1 -> Display3/1, Max Throttle Cable Stroke (mm)/1, Subtract1/1
  Product2/1 -> Display4/1, Subtract1/2, Throttle Cable Stroke (mm)/1
  Gain1/1 -> Product2/2
  Throttle Cable Tension (N)/1 -> Display/1, Product/1
  Subtract1/1 -> Display8/1, Throttle Cable Stroke Available/1

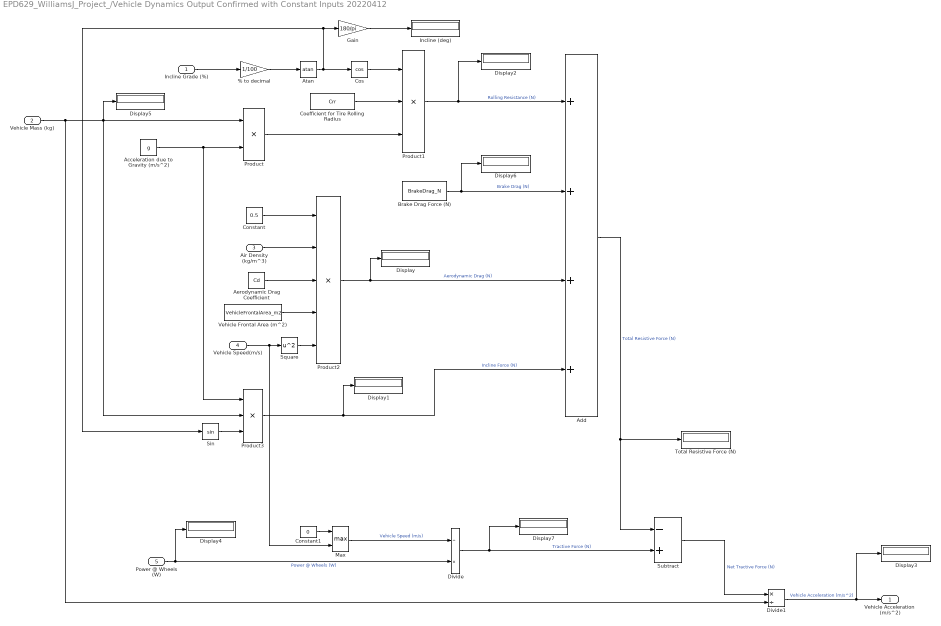
== system EPD629_WilliamsJ_Project_/Vehicle Dynamics Output Confirmed with Constant Inputs 20220412  ==
  Incline Grade (%) : Inport
  Vehicle Mass (kg) : Inport  Port=2
  Air Density (kg/m^3) : Inport  Port=3
  Vehicle Speed(m/s) : Inport  Port=4
  Power @ Wheels (W) : Inport  Port=5
  % to decimal : Gain  Gain=1/100
  Acceleration due to Gravity (m/s^2) : Constant  Value=g
  Add : Sum  Inputs=++++
  Aerodynamic Drag Coefficient : Constant  Value=Cd
  Atan : Trigonometry  Operator=atan
  Brake Drag Force (N) : Constant  Value=BrakeDrag_N
  Coefficient for Tire Rolling Radius : Constant  Value=Crr
  Constant : Constant  Value=0.5
  Constant1 : Constant  Value=0
  Cos : Trigonometry  Operator=cos
  Display{,1..7} (8 alike) : Display
  Divide : Product  Inputs=/*
  Divide1 : Product  Inputs=*/
  Gain : Gain  Gain=180/pi
  Incline (deg) : Display
  Max : MinMax  Function=max  Inputs=2
  Product : Product
  Product1 : Product  Inputs=3
  Product2 : Product  Inputs=5
  Product3 : Product  Inputs=3
  Sin : Trigonometry
  Square : Math  Operator=square  SaturateOnIntegerOverflow=on
  Subtract : Sum  Inputs=-+
  Total Resistive Force (N) : Display
  Vehicle Frontal Area (m^2) : Constant  Value=VehicleFrontalArea_m2
  Vehicle Acceleration (m/s^2) : Outport
  wires:
  Incline Grade (%)/1 -> % to decimal/1
  % to decimal/1 -> Atan/1
  Gain/1 -> Incline (deg)/1
  Atan/1 -> Sin/1, Gain/1, Cos/1
  Vehicle Mass (kg)/1 -> Display5/1, Product3/2, Product/1, Divide1/2
  Acceleration due to Gravity (m/s^2)/1 -> Product/2, Product3/1
  Cos/1 -> Product1/1
  Coefficient for Tire Rolling Radius/1 -> Product1/2
  Product/1 -> Product1/3
  Product1/1 -> Display2/1, Add/1  "Rolling Resistance (N)"
  Vehicle Speed(m/s)/1 -> Square/1, Max/2
  Constant/1 -> Product2/1
  Air Density (kg/m^3)/1 -> Product2/2
  Aerodynamic Drag Coefficient/1 -> Product2/3
  Vehicle Frontal Area (m^2)/1 -> Product2/4
  Square/1 -> Product2/5
  Product2/1 -> Add/3, Display/1  "Aerodynamic Drag (N)"
  Brake Drag Force (N)/1 -> Display6/1, Add/2  "Brake Drag (N)"
  Sin/1 -> Product3/3
  Product3/1 -> Display1/1, Add/4  "Incline Force (N)"
  Add/1 -> Total Resistive Force (N)/1, Subtract/1  "Total Resistive Force (N)"
  Power @ Wheels (W)/1 -> Display4/1, Divide/2  "Power @ Wheels (W)"
  Constant1/1 -> Max/1
  Max/1 -> Divide/1  "Vehicle Speed (m/s)"
  Divide/1 -> Display7/1, Subtract/2  "Tractive Force (N)"
  Subtract/1 -> Divide1/1  "Net Tractive Force (N)"
  Divide1/1 -> Display3/1, Vehicle Acceleration (m/s^2)/1  "Vehicle Acceleration (m/s^2)"
